simulink model "DCmodel_controlled_1_2020"  (R2020b)
settings: Solver=ode45  StartTime=0.0  StopTime=5  RelTol=1e-3
values from neighbouring files (symbols this model uses):
  degs2rpm = 0.166666666667    [DIGIT1-BE10.mat]    (also in DIGIT1-FE10.mat; DIGIT1-FE20.mat; DIGIT1-FE4.mat; DIGIT1-TR10.mat)
  denF = [1 0.515887399724 0.219018124689]    [DIGIT1-BE10.mat]    (also in DIGIT1-FE10.mat; DIGIT1-FE20.mat = [1 1.15847990004 0.419704605826]; DIGIT1-FE4.mat = [1 -0.53010968182 0.221694090774]; DIGIT1-TR10.mat)
  drv =     [DIGIT1-BE10.mat]    (also in DIGIT1-FE10.mat; DIGIT1-FE20.mat; DIGIT1-FE4.mat; DIGIT1-TR10.mat)
  filt =     [DIGIT1-BE10.mat]    (also in DIGIT1-FE10.mat; DIGIT1-FE20.mat; DIGIT1-FE4.mat; DIGIT1-TR10.mat)
  gbox =     [DIGIT1-BE10.mat]    (also in DIGIT1-FE10.mat; DIGIT1-FE20.mat; DIGIT1-FE4.mat; DIGIT1-TR10.mat)
  mld =     [DIGIT1-BE10.mat]    (also in DIGIT1-FE10.mat; DIGIT1-FE20.mat; DIGIT1-FE4.mat; DIGIT1-TR10.mat)
  mot =     [DIGIT1-BE10.mat]    (also in DIGIT1-FE10.mat; DIGIT1-FE20.mat; DIGIT1-FE4.mat; DIGIT1-TR10.mat)
  numF = [86.7452762207 0 -86.7452762207]    [DIGIT1-BE10.mat]    (also in DIGIT1-FE10.mat; DIGIT1-FE20.mat = [64.4546126467 0 -64.4546126467]; DIGIT1-FE4.mat = [86.4480511192 0 -86.4480511192]; DIGIT1-TR10.mat)
  rads2rpm = 9.54929658551    [DIGIT1-BE10.mat]    (also in DIGIT1-FE10.mat; DIGIT1-FE20.mat; DIGIT1-FE4.mat; DIGIT1-TR10.mat)
  rpm2rads = 0.10471975512    [DIGIT1-BE10.mat]    (also in DIGIT1-FE10.mat; DIGIT1-FE20.mat; DIGIT1-FE4.mat; DIGIT1-TR10.mat)
  sens =     [DIGIT1-BE10.mat]    (also in DIGIT1-FE10.mat; DIGIT1-FE20.mat; DIGIT1-FE4.mat; DIGIT1-TR10.mat)
  Ts = 0.01    [DIGIT1-BE10.mat]    (also in DIGIT1-FE10.mat; DIGIT1-FE20.mat = 0.02; DIGIT1-FE4.mat = 0.004; DIGIT1-TR10.mat)
undefined symbols (not defined in the file or in its folder): DiscIntNeverNeededParam
settings Model: Creator=emanuelevitetta  LastModifiedBy=emanuelevitetta
settings SolverCC: ZeroCrossAlgorithm=Adaptive
settings DebuggingCC: IgnoredZcDiagnostic=none  SFMachineParentedDataDiag=error

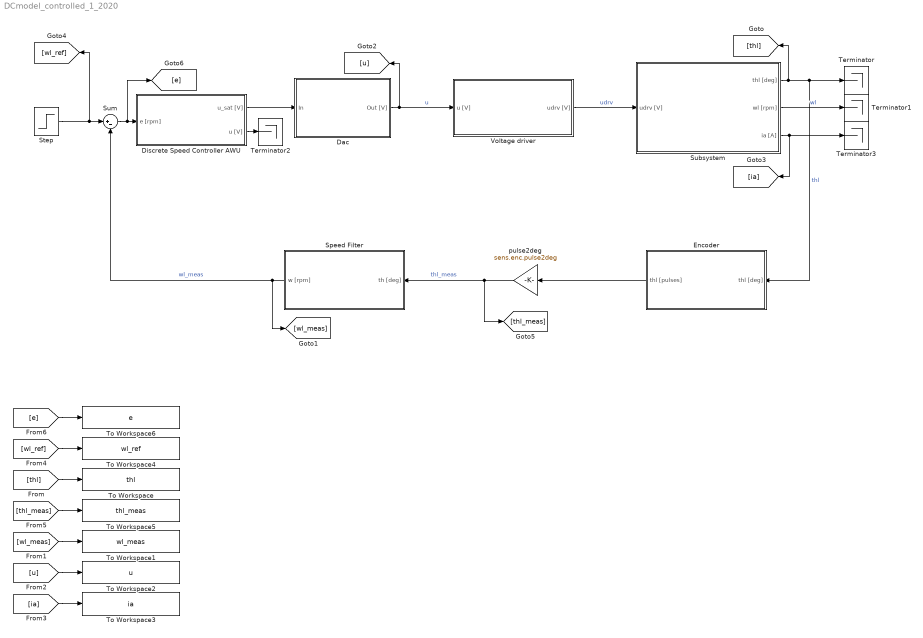
== system DCmodel_controlled_1_2020 ==
  Dac : Subsystem
  Discrete Speed Controller AWU : Subsystem
  Encoder : Subsystem
  Speed Filter : Subsystem
  Step : Step  After=250  SampleTime=0
  Subsystem : Subsystem
  Sum : Sum  Inputs=|+-
  Terminator{,1..3} (4 alike) : Terminator
  To Workspace : ToWorkspace  VariableName=thl  SaveFormat=Timeseries  SampleTime=-1
      settings: Save2DSignal=2-D array (concatenate along first dimension)
  To Workspace1 : ToWorkspace  VariableName=wl_meas  SaveFormat=Timeseries  SampleTime=-1
      settings: Save2DSignal=2-D array (concatenate along first dimension)
  To Workspace2 : ToWorkspace  VariableName=u  SaveFormat=Timeseries  SampleTime=-1
      settings: Save2DSignal=2-D array (concatenate along first dimension)
  To Workspace3 : ToWorkspace  VariableName=ia  SaveFormat=Timeseries  SampleTime=-1
      settings: Save2DSignal=2-D array (concatenate along first dimension)
  To Workspace4 : ToWorkspace  VariableName=wl_ref  SaveFormat=Timeseries  SampleTime=-1
      settings: Save2DSignal=2-D array (concatenate along first dimension)
  To Workspace5 : ToWorkspace  VariableName=thl_meas  SaveFormat=Timeseries  SampleTime=-1
      settings: Save2DSignal=2-D array (concatenate along first dimension)
  To Workspace6 : ToWorkspace  VariableName=e  SaveFormat=Timeseries  SampleTime=-1
      settings: Save2DSignal=2-D array (concatenate along first dimension)
  Voltage driver : Subsystem
  pulse2deg : Gain  Gain=sens.enc.pulse2deg
  wires:
  Dac/1(Out [V]) -> [u], Voltage driver/1(u [V])  "u"
  Encoder/1(thl [pulses]) -> pulse2deg/1
  Voltage driver/1(udrv [V]) -> Subsystem/1(udrv [V])  "udrv"
  Subsystem/2(wl [rpm]) -> Terminator1/1  "wl"
  Subsystem/1(thl [deg]) -> Terminator/1, Encoder/1(thl [deg]), [thl]  "thl"
  pulse2deg/1 -> [thl_meas], Speed Filter/1(th [deg])  "thl_meas"
  Speed Filter/1(w [rpm]) -> Sum/2, [wl_meas]  "wl_meas"
  Subsystem/3(ia [A]) -> Terminator3/1, [ia]
  [thl] -> To Workspace/1
  [wl_meas] -> To Workspace1/1
  [ia] -> To Workspace3/1
  [u] -> To Workspace2/1
  [wl_ref] -> To Workspace4/1
  [thl_meas] -> To Workspace5/1
  Sum/1 -> [e], Discrete Speed Controller AWU/1(e [rpm])
  Discrete Speed Controller AWU/1(u_sat [V]) -> Dac/1(In)
  [e] -> To Workspace6/1
  Step/1 -> [wl_ref], Sum/1
  Discrete Speed Controller AWU/2(u [V]) -> Terminator2/1

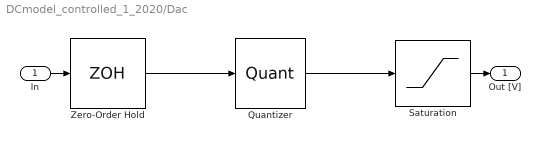
== system DCmodel_controlled_1_2020/Dac ==
  In : Inport
  Quantizer : Quantizer  QuantizationInterval=daq.dac.q
  Saturation : Saturate  UpperLimit=10  LowerLimit=-10
  Zero-Order Hold : ZeroOrderHold  SampleTime=0.001
  Out [V] : Outport
  wires:
  In/1 -> Zero-Order Hold/1
  Zero-Order Hold/1 -> Quantizer/1
  Saturation/1 -> Out [V]/1
  Quantizer/1 -> Saturation/1

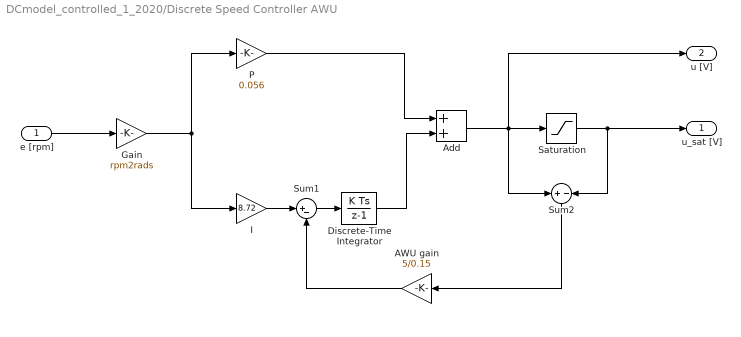
== system DCmodel_controlled_1_2020/Discrete Speed Controller AWU ==
  e [rpm] : Inport
  AWU gain : Gain  Gain=5/0.15
  Add : Sum
  Discrete-Time Integrator : DiscreteIntegrator  SampleTime=Ts  ICPrevOutput=DiscIntNeverNeededParam  ICPrevScaledInput=DiscIntNeverNeededParam
  Gain : Gain  Gain=rpm2rads
  I : Gain  Gain=8.72
  P : Gain  Gain=0.056
  Saturation : Saturate  UpperLimit=10  LowerLimit=-10
  Sum1 : Sum  Inputs=|+-
  Sum2 : Sum  Inputs=+-
  u_sat [V] : Outport
  u [V] : Outport  Port=2
  wires:
  e [rpm]/1 -> Gain/1
  P/1 -> Add/1
  Add/1 -> u [V]/1, Sum2/1, Saturation/1
  Saturation/1 -> Sum2/2, u_sat [V]/1
  Gain/1 -> I/1, P/1
  Sum1/1 -> Discrete-Time Integrator/1
  I/1 -> Sum1/1
  AWU gain/1 -> Sum1/2
  Sum2/1 -> AWU gain/1
  Discrete-Time Integrator/1 -> Add/2

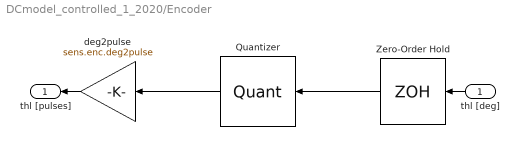
== system DCmodel_controlled_1_2020/Encoder ==
  thl [deg] : Inport
  Quantizer : Quantizer  QuantizationInterval=sens.enc.pulse2deg
  Zero-Order Hold : ZeroOrderHold  SampleTime=0.001
  deg2pulse : Gain  Gain=sens.enc.deg2pulse
  thl [pulses] : Outport
  wires:
  deg2pulse/1 -> thl [pulses]/1
  Quantizer/1 -> deg2pulse/1
  thl [deg]/1 -> Zero-Order Hold/1
  Zero-Order Hold/1 -> Quantizer/1

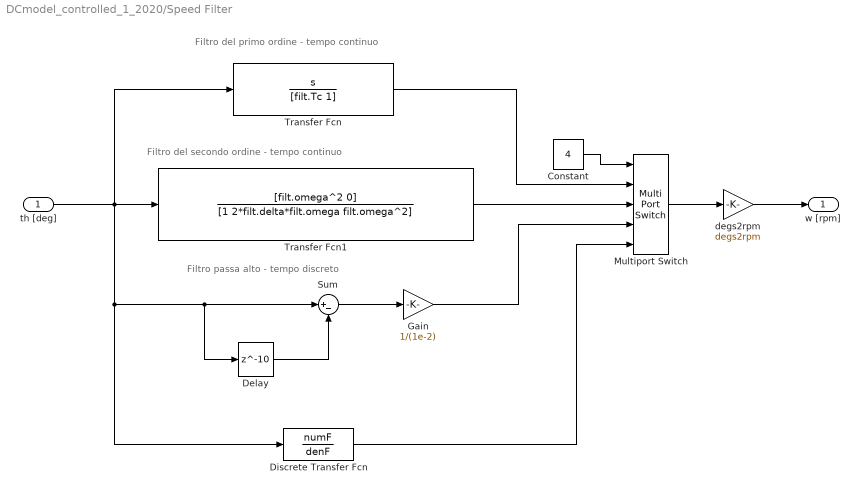
== system DCmodel_controlled_1_2020/Speed Filter ==
  note: Filtro passa alto - tempo discreto
  note: Filtro del secondo ordine - tempo continuo
  note: Filtro del primo ordine - tempo continuo
  th [deg] : Inport
  Constant : Constant  Value=4
  Delay : Delay  DelayLength=10  InitialCondition=0
  Discrete Transfer Fcn : DiscreteTransferFcn  Numerator=numF  Denominator=denF  SampleTime=Ts
  Gain : Gain  Gain=1/(1e-2)
  Multiport Switch : MultiPortSwitch  Inputs=4
  Sum : Sum  Inputs=|+-
  Transfer Fcn : TransferFcn  Numerator=[1 0]  Denominator=[filt.Tc 1]
  Transfer Fcn1 : TransferFcn  Numerator=[filt.omega^2 0]  Denominator=[1 2*filt.delta*filt.omega filt.omega^2]
  degs2rpm : Gain  Gain=degs2rpm
  w [rpm] : Outport
  wires:
  degs2rpm/1 -> w [rpm]/1
  Transfer Fcn1/1 -> Multiport Switch/3
  Multiport Switch/1 -> degs2rpm/1
  Gain/1 -> Multiport Switch/4
  Delay/1 -> Sum/2
  Sum/1 -> Gain/1
  Constant/1 -> Multiport Switch/1
  Transfer Fcn/1 -> Multiport Switch/2
  th [deg]/1 -> Discrete Transfer Fcn/1, Delay/1, Sum/1, Transfer Fcn/1, Transfer Fcn1/1
  Discrete Transfer Fcn/1 -> Multiport Switch/5

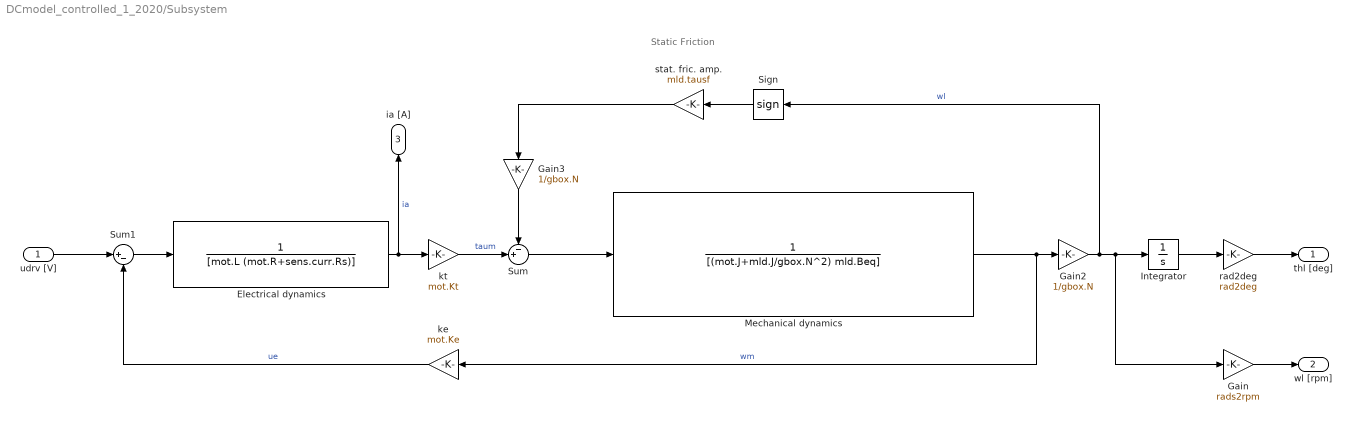
== system DCmodel_controlled_1_2020/Subsystem ==
  note: Static Friction
  udrv [V] : Inport
  Electrical dynamics : TransferFcn  Denominator=[mot.L (mot.R+sens.curr.Rs)]
  Gain : Gain  Gain=rads2rpm
  Gain2 : Gain  Gain=1/gbox.N
  Gain3 : Gain  Gain=1/gbox.N
  Integrator : Integrator
  Mechanical dynamics : TransferFcn  Denominator=[(mot.J+mld.J/gbox.N^2) mld.Beq]
  Sign : Signum
  Sum : Sum  Inputs=-+|
  Sum1 : Sum  Inputs=|+-
  ke : Gain  Gain=mot.Ke
  kt : Gain  Gain=mot.Kt
  rad2deg : Gain  Gain=rad2deg
  stat. fric. amp. : Gain  Gain=mld.tausf
  thl [deg] : Outport
  wl [rpm] : Outport  Port=2
  ia [A] : Outport  Port=3
  wires:
  rad2deg/1 -> thl [deg]/1
  Integrator/1 -> rad2deg/1
  Gain/1 -> wl [rpm]/1
  kt/1 -> Sum/2  "taum"
  Sum/1 -> Mechanical dynamics/1
  Electrical dynamics/1 -> kt/1, ia [A]/1  "ia"
  Mechanical dynamics/1 -> ke/1, Gain2/1  "wm"
  Gain2/1 -> Sign/1, Gain/1, Integrator/1  "wl"
  Sign/1 -> stat. fric. amp./1
  stat. fric. amp./1 -> Gain3/1
  Sum1/1 -> Electrical dynamics/1
  ke/1 -> Sum1/2  "ue"
  udrv [V]/1 -> Sum1/1
  Gain3/1 -> Sum/1

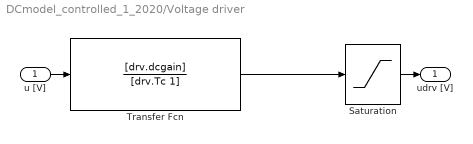
== system DCmodel_controlled_1_2020/Voltage driver ==
  u [V] : Inport
  Saturation : Saturate  UpperLimit=12  LowerLimit=-12
  Transfer Fcn : TransferFcn  Numerator=[drv.dcgain]  Denominator=[drv.Tc 1]
  udrv [V] : Outport
  wires:
  u [V]/1 -> Transfer Fcn/1
  Saturation/1 -> udrv [V]/1
  Transfer Fcn/1 -> Saturation/1
